simulink model "other_final_model"  (R2024a)
settings: Solver=VariableStepAuto  StartTime=0.0  StopTime=10.0  RelTol=1e-3
values from neighbouring files (symbols this model uses):
  C1_LUT = [1913.6,12447,30609 ... (first row only)    [data_thermal.m]
  C2_LUT = [1913.6,12447,30609 ... (first row only)    [data_thermal.m]
  Capacity_LUT = [28.01,27.63,27.64]    [data_thermal.m]
  Em_LUT = [3.49,3.51,3.52;3.55,3.56,3.56 ... (first row only)    [data_thermal.m]
  R0_LUT = [0.0117,0.0085,0.0090;0.0110,0.0085,0.0090 ... (first row only)    [data_thermal.m]
  R1_LUT = [0.0109,0.0029,0.0013;0.0069,0.0024,0.0012 ... (first row only)    [data_thermal.m]
  R2_LUT = [0.0109,0.0029,0.0013;0.0069,0.0024,0.0012 ... (first row only)    [data_thermal.m]
  SOC_LUT = [0;0.100;0.250;0.500;0.750;0.900;1.00]    [data_thermal.m]
  Temperature_LUT = [278.15,293.15,313.15]    [data_thermal.m]
settings Model: Creator=ACER  LastModifiedBy=ACER

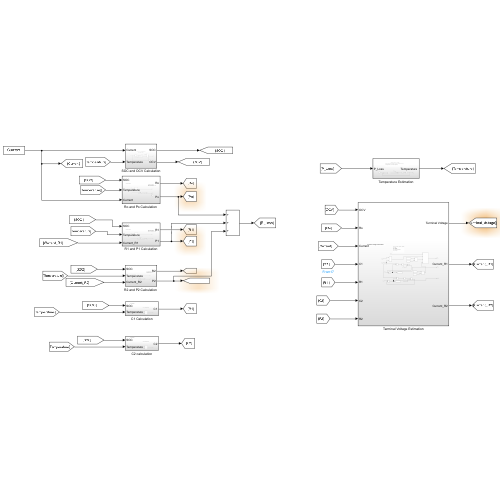
[thumbnail: Simulink's stored preview of the top-level diagram]
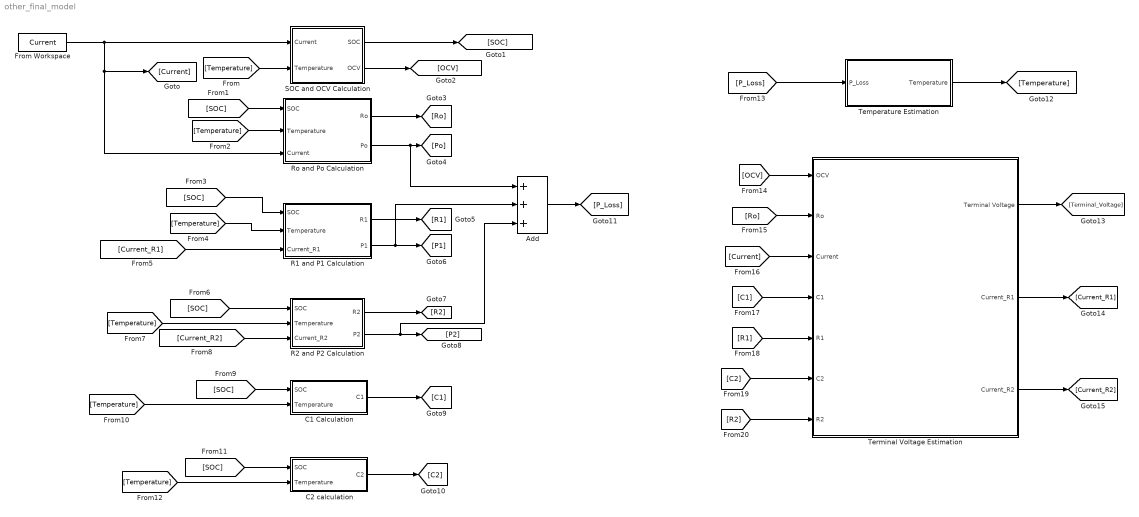
== system other_final_model ==
  Add : Sum  Inputs=+++
  C1 Calculation : Subsystem
  C2 calculation : Subsystem
  From Workspace : FromWorkspace  VariableName=Current
  R1 and P1 Calculation : Subsystem
  "R2 and P2 Calculation " : Subsystem
  "Ro and Po Calculation " : Subsystem
  SOC and OCV Calculation : Subsystem
  Temperature Estimation : Subsystem
  Terminal Voltage Estimation : Subsystem
  wires:
  "Ro and Po Calculation "/1(Ro) -> [Ro]
  [Temperature] -> C1 Calculation/2("Temperature ")
  [SOC] -> "Ro and Po Calculation "/1(SOC)
  "R2 and P2 Calculation "/1(R2) -> [R2]
  R1 and P1 Calculation/2(P1) -> Add/2, [P1]
  SOC and OCV Calculation/1(SOC) -> [SOC]
  [Temperature] -> SOC and OCV Calculation/2("Temperature ")
  R1 and P1 Calculation/1(R1) -> [R1]
  Add/1 -> [P_Loss]
  [Temperature] -> R1 and P1 Calculation/2("Temperature ")
  [Current_R1] -> R1 and P1 Calculation/3("Current_R1 ")
  "Ro and Po Calculation "/2(Po) -> Add/1, [Po]
  "R2 and P2 Calculation "/2(P2) -> Add/3, [P2]
  [SOC] -> R1 and P1 Calculation/1(SOC)
  [SOC] -> C1 Calculation/1(SOC)
  [SOC] -> C2 calculation/1(SOC)
  C1 Calculation/1(C1) -> [C1]
  [SOC] -> "R2 and P2 Calculation "/1(SOC)
  [Current_R2] -> "R2 and P2 Calculation "/3("Current_R2 ")
  [Temperature] -> "R2 and P2 Calculation "/2("Temperature ")
  [Temperature] -> "Ro and Po Calculation "/2("Temperature ")
  C2 calculation/1(C2) -> [C2]
  [Temperature] -> C2 calculation/2("Temperature ")
  SOC and OCV Calculation/2(OCV) -> [OCV]
  [P_Loss] -> Temperature Estimation/1(P_Loss)
  Temperature Estimation/1("Temperature ") -> [Temperature]
  [OCV] -> Terminal Voltage Estimation/1(OCV)
  [Ro] -> Terminal Voltage Estimation/2(Ro)
  [Current] -> Terminal Voltage Estimation/3("Current ")
  [C1] -> Terminal Voltage Estimation/4(C1)
  [R1] -> Terminal Voltage Estimation/5(R1)
  [C2] -> Terminal Voltage Estimation/6(C2)
  [R2] -> Terminal Voltage Estimation/7(R2)
  Terminal Voltage Estimation/1(Terminal Voltage) -> [Terminal_Voltage]
  Terminal Voltage Estimation/2(Current_R1) -> [Current_R1]
  Terminal Voltage Estimation/3(Current_R2) -> [Current_R2]
  From Workspace/1 -> "Ro and Po Calculation "/3("Current "), [Current], SOC and OCV Calculation/1("Current ")

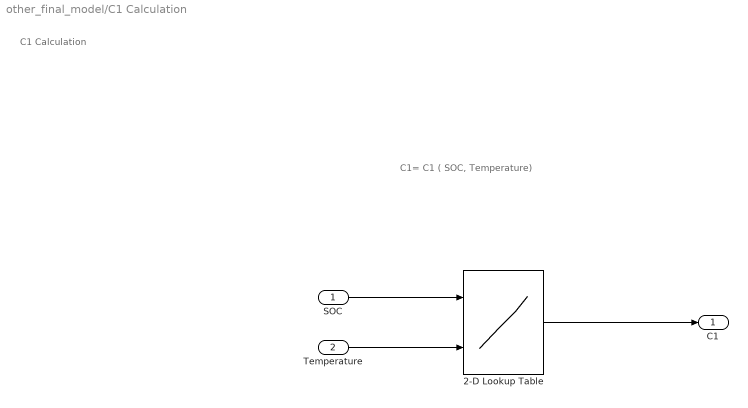
== system other_final_model/C1 Calculation ==
  note: C1 Calculation
  note: C1= C1 ( SOC, Temperature)
  SOC : Inport
  "Temperature " : Inport  Port=2
  2-D Lookup Table : Lookup_n-D  BreakpointsForDimension1=SOC_LUT  BreakpointsForDimension2=Temperature_LUT  Table=C1_LUT  InternalRulePriority=Speed  RndMeth=Simplest
      settings: InputPortMap=u0,u1
  C1 : Outport
  wires:
  2-D Lookup Table/1 -> C1/1
  SOC/1 -> 2-D Lookup Table/1
  "Temperature "/1 -> 2-D Lookup Table/2

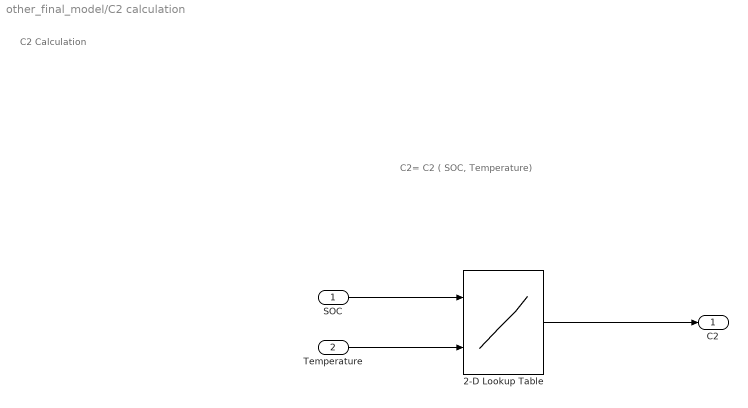
== system other_final_model/C2 calculation ==
  note: C2= C2 ( SOC, Temperature)
  note: C2 Calculation
  SOC : Inport
  "Temperature " : Inport  Port=2
  2-D Lookup Table : Lookup_n-D  BreakpointsForDimension1=SOC_LUT  BreakpointsForDimension2=Temperature_LUT  Table=C2_LUT  InternalRulePriority=Speed  RndMeth=Simplest
      settings: InputPortMap=u0,u1
  C2 : Outport
  wires:
  SOC/1 -> 2-D Lookup Table/1
  2-D Lookup Table/1 -> C2/1
  "Temperature "/1 -> 2-D Lookup Table/2

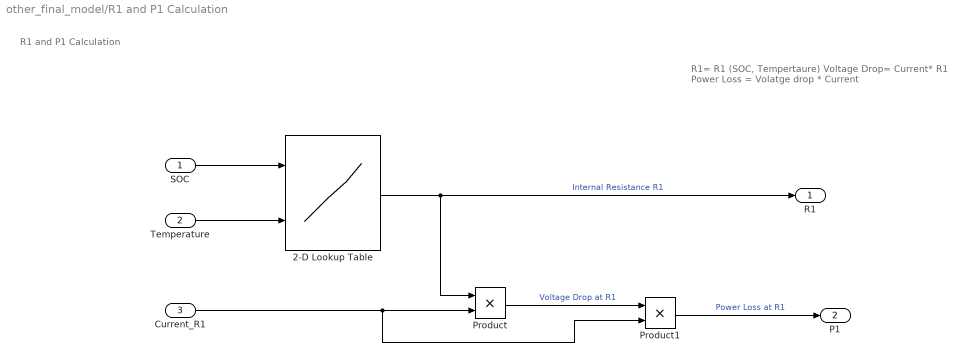
== system other_final_model/R1 and P1 Calculation ==
  note: R1= R1 (SOC, Tempertaure)
      | Voltage Drop= Current* R1
      | Power Loss = Volatge drop * Current
  note: R1 and P1 Calculation
  SOC : Inport
  "Temperature " : Inport  Port=2
  "Current_R1 " : Inport  Port=3
  2-D Lookup Table : Lookup_n-D  BreakpointsForDimension1=SOC_LUT  BreakpointsForDimension2=Temperature_LUT  Table=R1_LUT  InternalRulePriority=Speed  RndMeth=Simplest
      settings: InputPortMap=u0,u1
  Product : Product
  Product1 : Product
  R1 : Outport
  P1 : Outport  Port=2
  wires:
  SOC/1 -> 2-D Lookup Table/1
  Product1/1 -> P1/1  "Power Loss at R1"
  2-D Lookup Table/1 -> R1/1, Product/1  "Internal Resistance R1"
  "Temperature "/1 -> 2-D Lookup Table/2
  "Current_R1 "/1 -> Product1/2, Product/2
  Product/1 -> Product1/1  "Voltage Drop at R1"

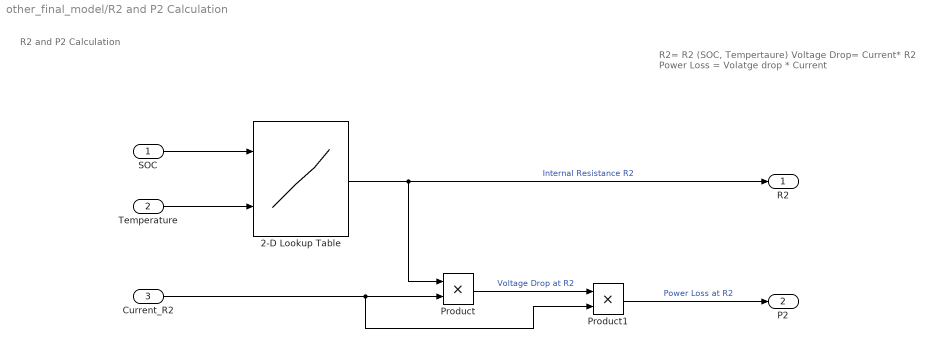
== system other_final_model/R2 and P2 Calculation  ==
  note: R2 and P2 Calculation
  note: R2= R2 (SOC, Tempertaure)
      | Voltage Drop= Current* R2
      | Power Loss = Volatge drop * Current
  SOC : Inport
  "Temperature " : Inport  Port=2
  "Current_R2 " : Inport  Port=3
  2-D Lookup Table : Lookup_n-D  BreakpointsForDimension1=SOC_LUT  BreakpointsForDimension2=Temperature_LUT  Table=R2_LUT  InternalRulePriority=Speed  RndMeth=Simplest
      settings: InputPortMap=u0,u1
  Product : Product
  Product1 : Product
  R2 : Outport
  P2 : Outport  Port=2
  wires:
  2-D Lookup Table/1 -> R2/1, Product/1  "Internal Resistance R2"
  Product1/1 -> P2/1  "Power Loss at R2"
  "Temperature "/1 -> 2-D Lookup Table/2
  SOC/1 -> 2-D Lookup Table/1
  "Current_R2 "/1 -> Product1/2, Product/2
  Product/1 -> Product1/1  "Voltage Drop at R2"

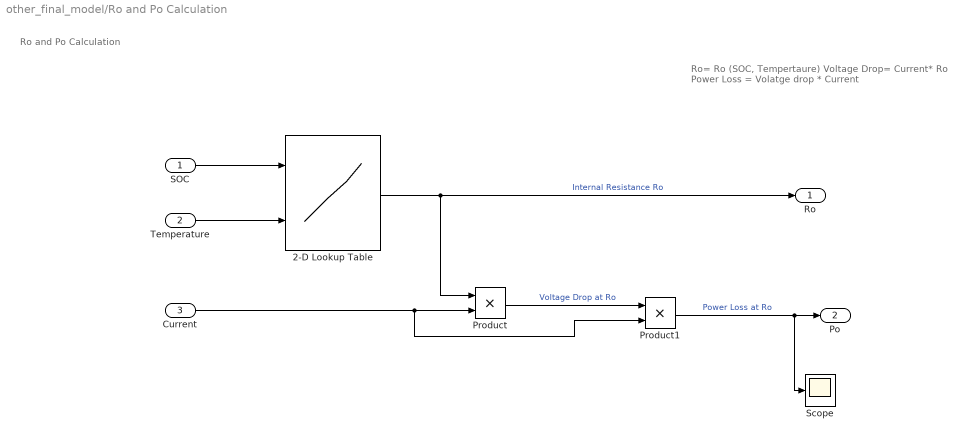
== system other_final_model/Ro and Po Calculation  ==
  note: Ro= Ro (SOC, Tempertaure)
      | Voltage Drop= Current* Ro
      | Power Loss = Volatge drop * Current
  note: Ro and Po Calculation
  SOC : Inport
  "Temperature " : Inport  Port=2
  "Current " : Inport  Port=3
  2-D Lookup Table : Lookup_n-D  BreakpointsForDimension1=SOC_LUT  BreakpointsForDimension2=Temperature_LUT  Table=R0_LUT  InternalRulePriority=Speed  RndMeth=Simplest
      settings: InputPortMap=u0,u1
  Product : Product
  Product1 : Product
  Scope : Scope
  Ro : Outport
  Po : Outport  Port=2
  wires:
  Product1/1 -> Scope/1, Po/1  "Power Loss at Ro"
  2-D Lookup Table/1 -> Ro/1, Product/1  "Internal Resistance Ro"
  "Temperature "/1 -> 2-D Lookup Table/2
  "Current "/1 -> Product1/2, Product/2
  SOC/1 -> 2-D Lookup Table/1
  Product/1 -> Product1/1  "Voltage Drop at Ro"

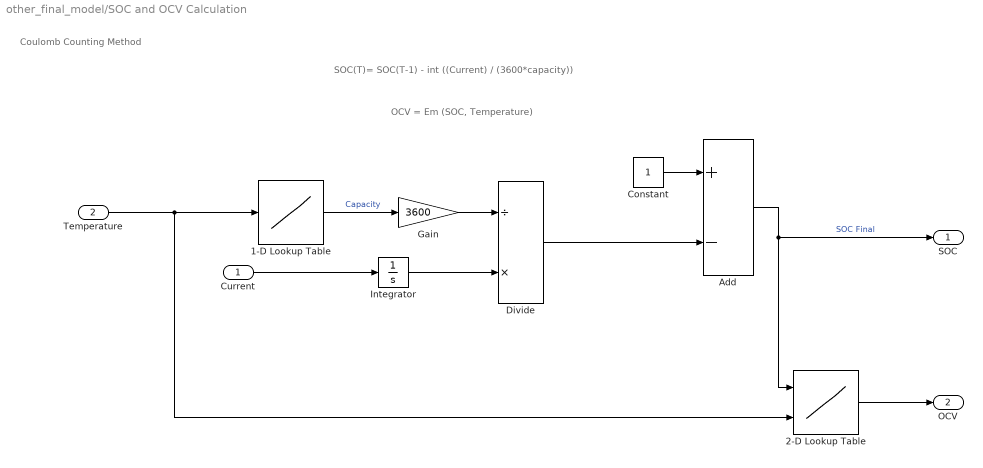
== system other_final_model/SOC and OCV Calculation ==
  note: Coulomb Counting Method
  note: OCV = Em (SOC, Temperature)
  note: SOC(T)= SOC(T-1) - int ((Current) / (3600*capacity))
  "Current " : Inport
  "Temperature " : Inport  Port=2
  1-D Lookup Table : Lookup_n-D  NumberOfTableDimensions=1  BreakpointsForDimension1=Temperature_LUT  Table=Capacity_LUT  InternalRulePriority=Speed  RndMeth=Simplest
  2-D Lookup Table : Lookup_n-D  BreakpointsForDimension1=SOC_LUT  BreakpointsForDimension2=Temperature_LUT  Table=Em_LUT  InternalRulePriority=Speed  RndMeth=Simplest
      settings: InputPortMap=u0,u1
  Add : Sum  Inputs=+-
  Constant : Constant
  Divide : Product  Inputs=/*
  Gain : Gain  Gain=3600
  Integrator : Integrator
  SOC : Outport
  OCV : Outport  Port=2
  wires:
  Integrator/1 -> Divide/2
  "Current "/1 -> Integrator/1
  1-D Lookup Table/1 -> Gain/1  "Capacity"
  Add/1 -> SOC/1, 2-D Lookup Table/1  "SOC Final"
  Gain/1 -> Divide/1
  Divide/1 -> Add/2
  "Temperature "/1 -> 2-D Lookup Table/2, 1-D Lookup Table/1
  Constant/1 -> Add/1
  2-D Lookup Table/1 -> OCV/1

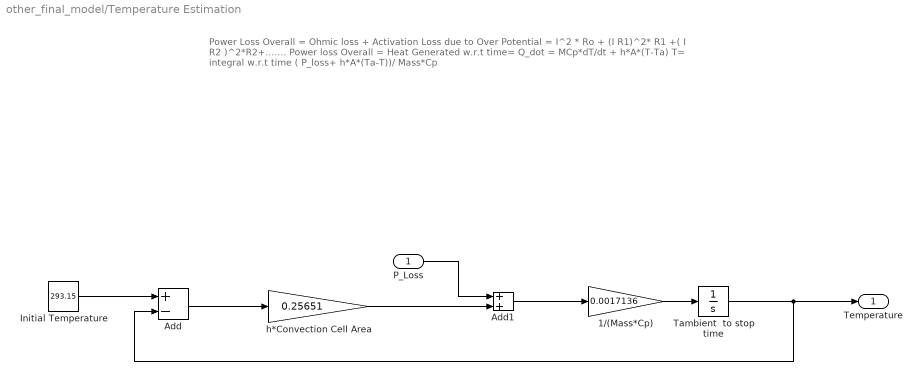
== system other_final_model/Temperature Estimation ==
  note: Power Loss Overall = Ohmic loss + Activation Loss due to Over Potential
      | = I^2 * Ro + (I R1)^2* R1 +( I R2 )^2*R2+.......
      |
      | Power loss Overall = Heat Generated w.r.t time= Q_dot = MCp*dT/dt + h*A*(T-Ta)
      |
      | T= integral w.r.t time ( P_loss+ h*A*(Ta-T))/ Mass*Cp
  P_Loss : Inport
  1/(Mass*Cp) : Gain  Gain=0.0017136
  Add : Sum  Inputs=+-
  Add1 : Sum
  "Initial Temperature " : Constant  Value=293.15
  Tambient  to stop time : Integrator  InitialCondition=293.15
  "h*Convection Cell Area " : Gain  Gain=0.25651
  "Temperature " : Outport
  wires:
  Tambient  to stop time/1 -> "Temperature "/1, Add/2
  "h*Convection Cell Area "/1 -> Add1/2
  Add/1 -> "h*Convection Cell Area "/1
  "Initial Temperature "/1 -> Add/1
  Add1/1 -> 1/(Mass*Cp)/1
  P_Loss/1 -> Add1/1
  1/(Mass*Cp)/1 -> Tambient  to stop time/1

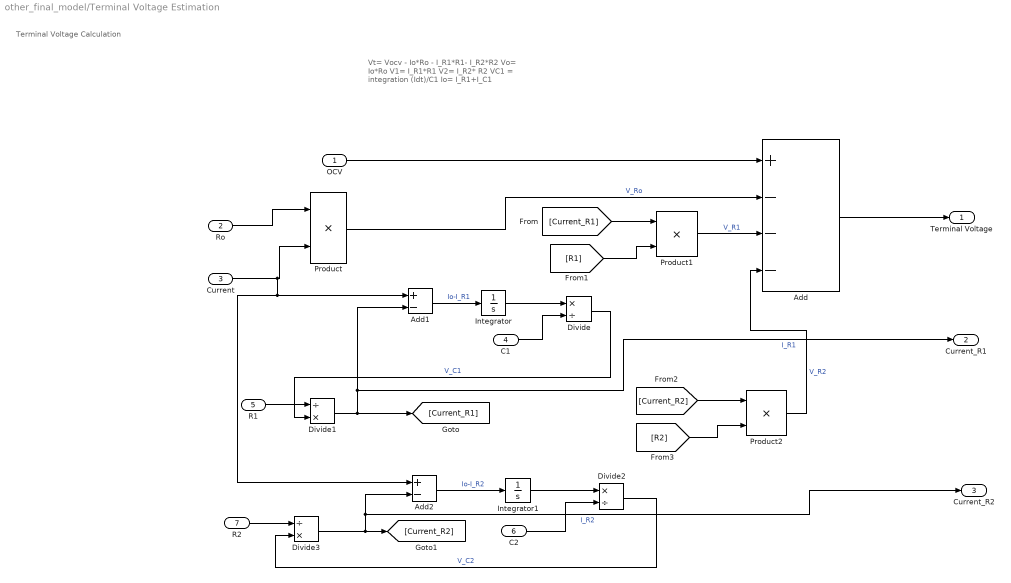
== system other_final_model/Terminal Voltage Estimation ==
  note: Vt= Vocv - Io*Ro - I_R1*R1- I_R2*R2
      | Vo= Io*Ro
      | V1= I_R1*R1
      | V2= I_R2* R2
      | VC1 = integration (Idt)/C1
      | Io= I_R1+I_C1
  note: Terminal Voltage Calculation
  OCV : Inport
  Ro : Inport  Port=2
  "Current " : Inport  Port=3
  C1 : Inport  Port=4
  R1 : Inport  Port=5
  C2 : Inport  Port=6
  R2 : Inport  Port=7
  Add : Sum  Inputs=+---
  Add1 : Sum  Inputs=+-
  Add2 : Sum  Inputs=+-
  Divide : Product  Inputs=*/
  Divide1 : Product  Inputs=/*
  Divide2 : Product  Inputs=*/
  Divide3 : Product  Inputs=/*
  Integrator : Integrator
  Integrator1 : Integrator
  Product : Product
  Product1 : Product
  Product2 : Product
  Terminal Voltage : Outport
  Current_R1 : Outport  Port=2
  Current_R2 : Outport  Port=3
  wires:
  Add/1 -> Terminal Voltage/1
  Integrator/1 -> Divide/1
  Integrator1/1 -> Divide2/1
  R1/1 -> Divide1/1
  Add1/1 -> Integrator/1  "Io-I_R1"
  C1/1 -> Divide/2
  Ro/1 -> Product/1
  OCV/1 -> Add/1
  [Current_R2] -> Product2/1
  "Current "/1 -> Add2/1, Add1/1, Product/2
  [R2] -> Product2/2
  Add2/1 -> Integrator1/1  "Io-I_R2"
  R2/1 -> Divide3/1
  [Current_R1] -> Product1/1
  Product1/1 -> Add/3  "V_R1"
  Product/1 -> Add/2  "V_Ro"
  Divide3/1 -> Current_R2/1, Add2/2, [Current_R2]  "I_R2"
  Divide2/1 -> Divide3/2  "V_C2"
  Divide1/1 -> Current_R1/1, Add1/2, [Current_R1]  "I_R1"
  [R1] -> Product1/2
  Divide/1 -> Divide1/2  "V_C1"
  Product2/1 -> Add/4  "V_R2"
  C2/1 -> Divide2/2
